simulink model "vrcrane_traj"  (Simulink 6.0)
settings: Solver=ode45  StartTime=0.0  StopTime=60  RelTol=1e-3
PostLoadFcn:
  | Ra=2.6;
  | La=0.012;
  | B=1e-1;
  | Kt=1e2;
  | Kv=3e-2;
  | Kg=1e-3;
  | J=0.1;
  | g=9.80665;
  | m_head=100;
  | Gamma=10;
undefined symbols (not defined in the file or in its folder): sigbuilder_block
libraries: simulink_extras x6, vrlib x6, simulink x1
settings Model: Creator=Danek  LastModifiedBy=Danek
settings DataIOCC: SignalLoggingName=logsOut
settings DebuggingCC: CheckExecutionContextPreStartOutputMsg=on  CheckExecutionContextRuntimeOutputMsg=on
settings ModelReferenceCC: UpdateModelReferenceTargets=IfOutOfDate
settings GRTTargetCC: LifeSpan=inf
settings SFSimCC: SFSimApplyToAllLibs=on  SFSimBuildMode=Incremental

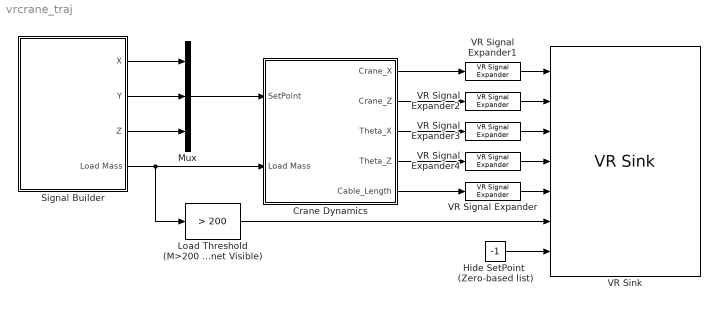
== system vrcrane_traj ==
  Crane Dynamics : Subsystem  EnableExecutionContextPropagation=on
  Hide SetPoint  (Zero-based list) : Constant  Value=-1
  Load Threshold (M>200 = Load on Magnet Visible) : simulink/Logic and Bit Operations/Compare To Constant  relop=>  const=200  LogicOutDataTypeMode=uint8
  Mux : Mux  Inputs=3
  Signal Builder : Subsystem  Tag=STV Subsys  LoadFcn=sigbuilder_block('load');  StartFcn=sigbuilder_block('start');  StopFcn=sigbuilder_block('stop');  ClipboardFcn=sigbuilder_block('clipboard');  EnableExecutionContextPropagation=on  mask(Sigbuilder block){}
      mask help: Sigbuilder GUI
      mask init:
      | if ~strcmp(get_param(bdroot(gcb),'SimulationStatus'),'stopped') tuvar = sigbuilder_block('maskInit'); end
      settings: CopyFcn=sigbuilder_block('copy');  DeleteFcn=sigbuilder_block('delete');  ModelCloseFcn=sigbuilder_block('modelClose');  PreSaveFcn=sigbuilder_block('preSave');  NameChangeFcn=sigbuilder_block('namechange');  OpenFcn=sigbuilder_block('open',[111.75 57.75 534.75 459.75 ]);  CloseFcn=sigbuilder_block('close');
      mask Display: plot(0,0,100,100,[10,10,40,40,10],[80,20,20,80,80],[40,10],[50,50], [40,27,10],[65,72,56],[40,25,25,10],[28,28,43,43]);
  VR Signal Expander : vrlib/VR Signal Expander  outwidth=3  outidx=[2]
  VR Signal Expander1 : vrlib/VR Signal Expander  outwidth=3  outidx=[1]
  VR Signal Expander2 : vrlib/VR Signal Expander  outwidth=3  outidx=[3]
  VR Signal Expander3 : vrlib/VR Signal Expander  outwidth=4  outidx=[4]
  VR Signal Expander4 : vrlib/VR Signal Expander  outwidth=4  outidx=[4]
  VR Sink : vrlib/VR Sink  SampleTime=0.1  ViewEnable=on  RemoteChange=off  RemoteView=off  FieldsWritten=Crane_X.translation.3.1.double#Crane_Z.translation.3.1.double#Parts_Rot_ZAxis.rotation.4.1.double#Parts_Rot_XAxis.rotation.4.1.double#CableUnit.scale.3.1.double#Load_Switch.whichChoice.1.1.double#SP_Highlight.whichChoice.1.1.double  WorldFileName=portal_crane.wrl  WorldDescription=VR Portal Crane  AutoView=on  FigureProperties="{'Position', 'Name', 'Viewpoint', 'CameraBound', 'CameraDirection', 'CameraPosition', 'CameraUpVector', 'ZoomFactor', 'Antialiasing', 'Headlight', 'Lighting', 'NavPanel', 'StatusBar', 'Textures', 'Transparency', 'Wireframe', 'NavZones', 'NavMode', 'NavSpeed', 'Record2DCompressMethod', 'Record2DCompressQuality', 'Record2D', 'Record2DFcn', 'Record2DFileName', 'Record2DStartFcn', 'Record2DStopFcn'; [1.3000000000000000e+001  7.8000000000000000e+001  5.7600000000000000e+002  3.8000000000000000e+002], 'VR Portal Crane', 'Overview', 'on', [-4.7942553860420378e-001  2.7565528915671302e-002 -8.7714952804505797e-001], [8.7686886571229490e+000 -3.9860053732208831e+000 -2.1939948026302826e+001], [3.4694469519536142e-017  9.9950656056293841e-001  3.1410752802896708e-002], [1.0000000000000000e+000], 'off', 'on', 'on', 'halfbar', 'on', 'on', 'on', 'off', 'off', 'examine', 'normal', 'auto', [7.5000000000000000e+001], 'off', 'vrrecordcallback(vrgcbf, ''Frame'');', '%f_anim_%n.avi', 'vrrecordcallback(vrgcbf, ''Start'');', 'vrrecordcallback(vrgcbf, ''Stop'');'}"
  wires:
  Crane Dynamics/5(Cable_Length) -> VR Signal Expander/1
  Crane Dynamics/1(Crane_X) -> VR Signal Expander1/1
  Crane Dynamics/3(Theta_X) -> VR Signal Expander3/1
  Crane Dynamics/2(Crane_Z) -> VR Signal Expander2/1
  Crane Dynamics/4(Theta_Z) -> VR Signal Expander4/1
  Mux/1 -> Crane Dynamics/1(SetPoint)
  Signal Builder/1(X) -> Mux/1
  Signal Builder/2(Y) -> Mux/2
  Signal Builder/3(Z) -> Mux/3
  Signal Builder/4(Load Mass) -> Crane Dynamics/2(Load Mass), Load Threshold (M>200 = Load on Magnet Visible)/1
  VR Signal Expander1/1 -> VR Sink/1
  VR Signal Expander2/1 -> VR Sink/2
  VR Signal Expander3/1 -> VR Sink/3
  VR Signal Expander4/1 -> VR Sink/4
  VR Signal Expander/1 -> VR Sink/5
  Load Threshold (M>200 = Load on Magnet Visible)/1 -> VR Sink/6
  Hide SetPoint  (Zero-based list)/1 -> VR Sink/7

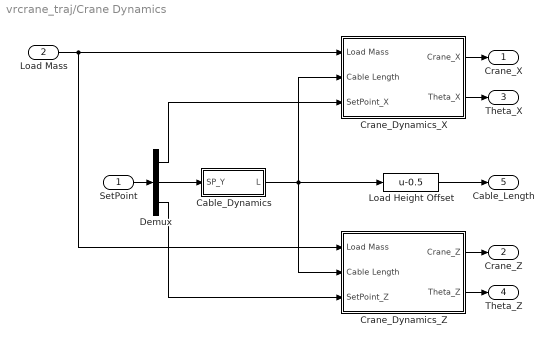
== system vrcrane_traj/Crane Dynamics ==
  SetPoint : Inport  LatchInput=off
  Load Mass : Inport  Port=2  LatchInput=off
  Cable_Dynamics : Subsystem  EnableExecutionContextPropagation=on
  Crane_Dynamics_X : Subsystem  EnableExecutionContextPropagation=on
  Crane_Dynamics_Z : Subsystem  EnableExecutionContextPropagation=on
  Demux : Demux  Outputs=3
  "Load Height Offset " : Fcn  Expr=u-0.5
  Crane_X : Outport
  Crane_Z : Outport  Port=2
  Theta_X : Outport  Port=3
  Theta_Z : Outport  Port=4
  Cable_Length : Outport  Port=5
  wires:
  Cable_Dynamics/1(L) -> Crane_Dynamics_X/2(Cable Length), Crane_Dynamics_Z/2(Cable Length), "Load Height Offset "/1
  Demux/2 -> Cable_Dynamics/1(SP_Y)
  Demux/1 -> Crane_Dynamics_X/3(SetPoint_X)
  Load Mass/1 -> Crane_Dynamics_Z/1(Load Mass), Crane_Dynamics_X/1(Load Mass)
  SetPoint/1 -> Demux/1
  Crane_Dynamics_X/1(Crane_X) -> Crane_X/1
  Crane_Dynamics_X/2(Theta_X) -> Theta_X/1
  "Load Height Offset "/1 -> Cable_Length/1
  Crane_Dynamics_Z/1(Crane_Z) -> Crane_Z/1
  Crane_Dynamics_Z/2(Theta_Z) -> Theta_Z/1
  Demux/3 -> Crane_Dynamics_Z/3(SetPoint_Z)

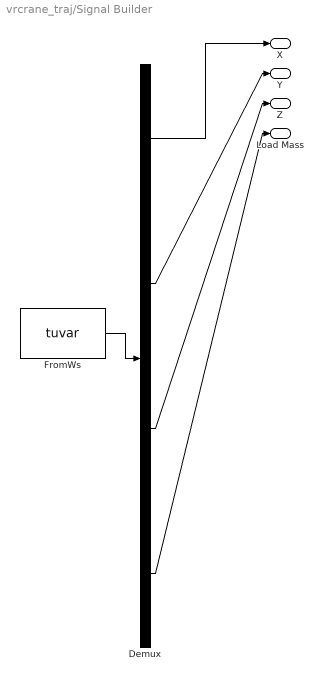
== system vrcrane_traj/Signal Builder ==
  Demux : Demux  Tag=STV Demux
  FromWs : FromWorkspace  Tag=STV FromWs  VariableName=tuvar  SampleTime=0  OutputAfterFinalValue=Holding final value  SigBuilderData=DataTag0  VnvData=DataTag1
      SigBuilderData=|
      | channels(1).label = 'X'
      | channels(1).allXData = {[0 17.9 17.9 34.9 34.9 35 36.8 36.8 60]}
      | channels(1).allYData = {[0 0 15 15 15.5 15 15 0 0]}
      | channels(2).label = 'Y'
      | channels(2).allXData = {[0 14 14 18 18 32 32 35 36.8 36.8 50 50 60]}
      | channels(2).allYData = {[4 4 0 0 4 4 0 0 0 4 4 0 0]}
      | channels(3).label = 'Z'
      | channels(3).allXData = {[0 3 3 18 18 34.9 35 37 37 60]}
      | channels(3).allYData = {[0 0 15 15 5 5 5 5 0 0]}
      | channels(4).label = 'Load Mass'
      | channels(4).allXData = {[0 17 17 36.2 36.2 60]}
      | channels(4).allYData = {[100 100 1000 1000 100 100]}
      | common.afterFinalStr = 'Hold final value'
      | common.sampleTime = 0
      | dataSet.timeRange = [0 60]
      | dataSet.name = 'Setpoint'
  X : Outport  Tag=STV Outport
  Y : Outport  Tag=STV Outport  Port=2
  Z : Outport  Tag=STV Outport  Port=3
  Load Mass : Outport  Tag=STV Outport  Port=4
  wires:
  Demux/1 -> X/1
  FromWs/1 -> Demux/1
  Demux/2 -> Y/1
  Demux/3 -> Z/1
  Demux/4 -> Load Mass/1

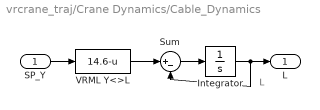
== system vrcrane_traj/Crane Dynamics/Cable_Dynamics ==
  note: L
  SP_Y : Inport  LatchInput=off
  Integrator : Integrator  InitialCondition=14.6  LimitOutput=on  UpperSaturationLimit=14.6  LowerSaturationLimit=4.6
  Sum : Sum  Inputs=|+-
  VRML Y<>L : Fcn  Expr=14.6-u
  L : Outport
  wires:
  Sum/1 -> Integrator/1
  VRML Y<>L/1 -> Sum/1
  Integrator/1 -> Sum/2, L/1
  SP_Y/1 -> VRML Y<>L/1

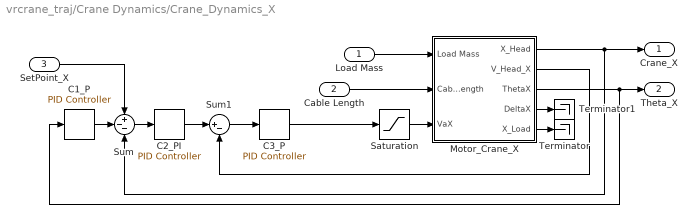
== system vrcrane_traj/Crane Dynamics/Crane_Dynamics_X ==
  Load Mass : Inport  LatchInput=off
  Cable Length : Inport  Port=2  LatchInput=off
  SetPoint_X : Inport  Port=3  LatchInput=off
  C1_P : simulink_extras/Additional Linear/PID Controller  P=-20  I=0  D=0
  C2_PI : simulink_extras/Additional Linear/PID Controller  P=2.5  I=0  D=0
  C3_P : simulink_extras/Additional Linear/PID Controller  P=5  I=0  D=0
  Motor_Crane_X : Subsystem  EnableExecutionContextPropagation=on
  Saturation : Saturate  UpperLimit=50  LowerLimit=-50
  Sum : Sum  Inputs=+--  SaturateOnIntegerOverflow=on  InputSameDT=on
  Sum1 : Sum  Inputs=|+-  SaturateOnIntegerOverflow=on  InputSameDT=on
  Terminator : Terminator
  Terminator1 : Terminator
  Crane_X : Outport
  Theta_X : Outport  Port=2
  wires:
  Motor_Crane_X/1(X_Head) -> Crane_X/1, Sum/3
  Load Mass/1 -> Motor_Crane_X/1(Load Mass)
  Motor_Crane_X/2(V_Head_X) -> Sum1/2
  Cable Length/1 -> Motor_Crane_X/2(Cable Length)
  Motor_Crane_X/3(ThetaX) -> Theta_X/1, C1_P/1
  Motor_Crane_X/4(DeltaX) -> Terminator1/1
  Motor_Crane_X/5(X_Load) -> Terminator/1
  SetPoint_X/1 -> Sum/1
  Sum/1 -> C2_PI/1
  C2_PI/1 -> Sum1/1
  Sum1/1 -> C3_P/1
  Saturation/1 -> Motor_Crane_X/3(VaX)
  C3_P/1 -> Saturation/1
  C1_P/1 -> Sum/2

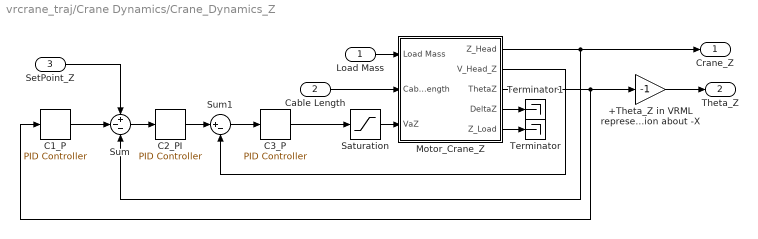
== system vrcrane_traj/Crane Dynamics/Crane_Dynamics_Z ==
  Load Mass : Inport  LatchInput=off
  Cable Length : Inport  Port=2  LatchInput=off
  SetPoint_Z : Inport  Port=3  LatchInput=off
  +Theta_Z in VRML represented by rotation about -X : Gain  Gain=-1
  C1_P : simulink_extras/Additional Linear/PID Controller  P=-20  I=0  D=0
  C2_PI : simulink_extras/Additional Linear/PID Controller  P=2.5  I=0  D=0
  C3_P : simulink_extras/Additional Linear/PID Controller  P=5  I=0  D=0
  Motor_Crane_Z : Subsystem  EnableExecutionContextPropagation=on
  Saturation : Saturate  UpperLimit=50  LowerLimit=-50
  Sum : Sum  Inputs=+--  SaturateOnIntegerOverflow=on  InputSameDT=on
  Sum1 : Sum  Inputs=|+-  SaturateOnIntegerOverflow=on  InputSameDT=on
  Terminator : Terminator
  Terminator1 : Terminator
  Crane_Z : Outport
  Theta_Z : Outport  Port=2
  wires:
  Motor_Crane_Z/1(Z_Head) -> Crane_Z/1, Sum/3
  Load Mass/1 -> Motor_Crane_Z/1(Load Mass)
  Cable Length/1 -> Motor_Crane_Z/2(Cable Length)
  Motor_Crane_Z/3(ThetaZ) -> +Theta_Z in VRML represented by rotation about -X/1, C1_P/1
  Motor_Crane_Z/4(DeltaZ) -> Terminator1/1
  Motor_Crane_Z/5(Z_Load) -> Terminator/1
  Saturation/1 -> Motor_Crane_Z/3(VaZ)
  C3_P/1 -> Saturation/1
  +Theta_Z in VRML represented by rotation about -X/1 -> Theta_Z/1
  Motor_Crane_Z/2(V_Head_Z) -> Sum1/2
  Sum/1 -> C2_PI/1
  C2_PI/1 -> Sum1/1
  Sum1/1 -> C3_P/1
  C1_P/1 -> Sum/2
  SetPoint_Z/1 -> Sum/1

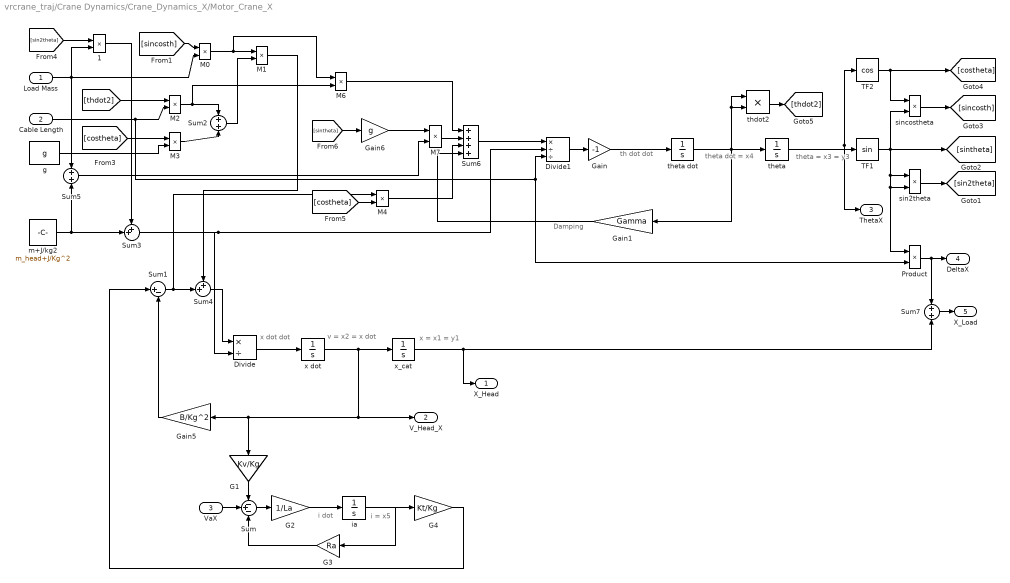
== system vrcrane_traj/Crane Dynamics/Crane_Dynamics_X/Motor_Crane_X ==
  note: i dot
  note: i = x5
  note: x = x1 = y1
  note: v = x2 = x dot
  note: theta = x3 = y3
  note: theta dot = x4
  note: x dot dot
  note: th dot dot
  note: Damping
  Load Mass : Inport  LatchInput=off
  Cable Length : Inport  Port=2  LatchInput=off
  VaX : Inport  Port=3  LatchInput=off
  " 1" : Product  Inputs=**  OutScaling=2^-10
  Divide : Product  Inputs=*/  OutScaling=2^-10
  Divide1 : Product  Inputs=*//  OutScaling=2^-10
  G1 : Gain  Orientation=down  Gain=Kv/Kg
  G2 : Gain  Gain=1/La
  G3 : Gain  Orientation=left  Gain=Ra
  G4 : Gain  Gain=Kt/Kg
  Gain : Gain  Gain=-1
  Gain1 : Gain  Orientation=left  Gain=Gamma
  Gain5 : Gain  Orientation=left  Gain=B/Kg^2
  Gain6 : Gain  Gain=g
  M{0..4,6..7} (7 alike) : Product  Inputs=**  OutScaling=2^-10
  Product : Product  SaturateOnIntegerOverflow=on
  Sum : Sum  Inputs=-+-
  Sum1 : Sum  Inputs=|+-
  Sum2 : Sum
  Sum3 : Sum  Inputs=++|
  Sum4 : Sum  Inputs=++|
  Sum5 : Sum
  Sum6 : Sum  Inputs=++++
  Sum7 : Sum
  TF1 : Trigonometry
  TF2 : Trigonometry  Operator=cos
  g : Constant  Value=g
  ia : Integrator
  m+J/kg2 : Constant  Value=m_head+J/Kg^2
  sin2theta : Product  Inputs=**  OutScaling=2^-10
  sincostheta : Product  Inputs=**  OutScaling=2^-10
  thdot2 : Product  Inputs=**  OutScaling=2^-10
  theta : Integrator
  theta dot : Integrator
  x dot : Integrator
  x_cat : Integrator
  X_Head : Outport
  V_Head_X : Outport  Port=2
  ThetaX : Outport  Port=3
  DeltaX : Outport  Port=4
  X_Load : Outport  Port=5
  wires:
  G1/1 -> Sum/1
  Sum/1 -> G2/1
  G2/1 -> ia/1
  ia/1 -> G3/1, G4/1
  G3/1 -> Sum/3
  x dot/1 -> x_cat/1, G1/1, Gain5/1, V_Head_X/1
  theta/1 -> ThetaX/1, TF1/1, TF2/1
  theta dot/1 -> theta/1, thdot2/2, thdot2/1, Gain1/1
  G4/1 -> Sum1/1
  Divide/1 -> x dot/1
  Gain5/1 -> Sum1/2
  sin2theta/1 -> [sin2theta]
  sincostheta/1 -> [sincosth]
  [sincosth] -> M0/1
  Load Mass/1 -> Sum5/1, M0/2, " 1"/2
  thdot2/1 -> [thdot2]
  M0/1 -> M1/1, M6/1
  [thdot2] -> M2/1
  [costheta] -> M3/1
  g/1 -> M3/2
  M3/1 -> Sum2/2
  Sum2/1 -> M1/2
  [sin2theta] -> " 1"/1
  " 1"/1 -> Sum3/1
  Sum3/1 -> Divide1/2, Divide/2
  Sum4/1 -> Divide/1
  M1/1 -> Sum4/1
  Sum1/1 -> Sum4/2, M4/1
  M2/1 -> Sum2/1, M6/2
  M6/1 -> Sum6/1
  [costheta] -> M4/2
  Sum5/1 -> M7/2
  [sintheta] -> Gain6/1
  Gain6/1 -> M7/1
  M7/1 -> Sum6/2
  M4/1 -> Sum6/3
  Sum6/1 -> Divide1/1
  Cable Length/1 -> M2/2, Divide1/3, Product/2
  Divide1/1 -> Gain/1
  Gain/1 -> theta dot/1
  x_cat/1 -> X_Head/1, Sum7/2
  VaX/1 -> Sum/2
  m+J/kg2/1 -> Sum3/2, Sum5/2
  Product/1 -> DeltaX/1, Sum7/1
  TF2/1 -> [costheta], sincostheta/1
  TF1/1 -> [sintheta], sincostheta/2, sin2theta/2, Product/1, sin2theta/1
  Sum7/1 -> X_Load/1
  Gain1/1 -> Sum6/4

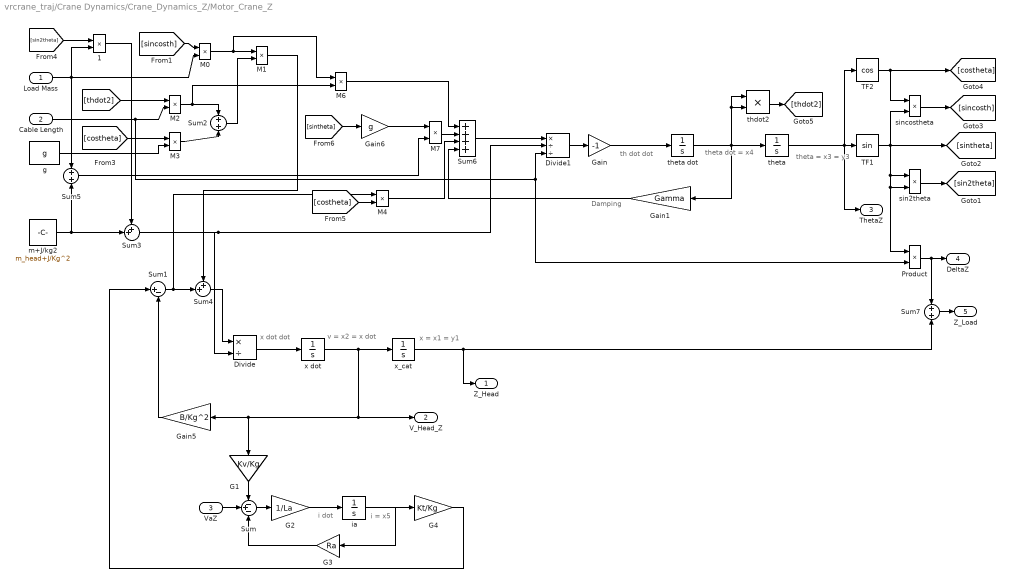
== system vrcrane_traj/Crane Dynamics/Crane_Dynamics_Z/Motor_Crane_Z ==
  note: i dot
  note: i = x5
  note: x = x1 = y1
  note: v = x2 = x dot
  note: theta = x3 = y3
  note: theta dot = x4
  note: x dot dot
  note: th dot dot
  note: Damping
  Load Mass : Inport  LatchInput=off
  Cable Length : Inport  Port=2  LatchInput=off
  VaZ : Inport  Port=3  LatchInput=off
  " 1" : Product  Inputs=**  OutScaling=2^-10
  Divide : Product  Inputs=*/  OutScaling=2^-10
  Divide1 : Product  Inputs=*//  OutScaling=2^-10
  G1 : Gain  Orientation=down  Gain=Kv/Kg
  G2 : Gain  Gain=1/La
  G3 : Gain  Orientation=left  Gain=Ra
  G4 : Gain  Gain=Kt/Kg
  Gain : Gain  Gain=-1
  Gain1 : Gain  Orientation=left  Gain=Gamma
  Gain5 : Gain  Orientation=left  Gain=B/Kg^2
  Gain6 : Gain  Gain=g
  M{0..4,6..7} (7 alike) : Product  Inputs=**  OutScaling=2^-10
  Product : Product  SaturateOnIntegerOverflow=on
  Sum : Sum  Inputs=-+-
  Sum1 : Sum  Inputs=|+-
  Sum2 : Sum
  Sum3 : Sum  Inputs=++|
  Sum4 : Sum  Inputs=++|
  Sum5 : Sum
  Sum6 : Sum  Inputs=++++
  Sum7 : Sum
  TF1 : Trigonometry
  TF2 : Trigonometry  Operator=cos
  g : Constant  Value=g
  ia : Integrator
  m+J/kg2 : Constant  Value=m_head+J/Kg^2
  sin2theta : Product  Inputs=**  OutScaling=2^-10
  sincostheta : Product  Inputs=**  OutScaling=2^-10
  thdot2 : Product  Inputs=**  OutScaling=2^-10
  theta : Integrator
  theta dot : Integrator
  x dot : Integrator
  x_cat : Integrator
  Z_Head : Outport
  V_Head_Z : Outport  Port=2
  ThetaZ : Outport  Port=3
  DeltaZ : Outport  Port=4
  Z_Load : Outport  Port=5
  wires:
  G1/1 -> Sum/1
  Sum/1 -> G2/1
  G2/1 -> ia/1
  ia/1 -> G3/1, G4/1
  G3/1 -> Sum/3
  x dot/1 -> x_cat/1, G1/1, Gain5/1, V_Head_Z/1
  theta/1 -> ThetaZ/1, TF1/1, TF2/1
  theta dot/1 -> theta/1, thdot2/2, thdot2/1, Gain1/1
  G4/1 -> Sum1/1
  Divide/1 -> x dot/1
  Gain5/1 -> Sum1/2
  sin2theta/1 -> [sin2theta]
  sincostheta/1 -> [sincosth]
  [sincosth] -> M0/1
  Load Mass/1 -> Sum5/1, M0/2, " 1"/2
  thdot2/1 -> [thdot2]
  M0/1 -> M1/1, M6/1
  [thdot2] -> M2/1
  [costheta] -> M3/1
  g/1 -> M3/2
  M3/1 -> Sum2/2
  Sum2/1 -> M1/2
  [sin2theta] -> " 1"/1
  " 1"/1 -> Sum3/1
  Sum3/1 -> Divide1/2, Divide/2
  Sum4/1 -> Divide/1
  M1/1 -> Sum4/1
  Sum1/1 -> Sum4/2, M4/1
  M2/1 -> Sum2/1, M6/2
  M6/1 -> Sum6/1
  [costheta] -> M4/2
  Sum5/1 -> M7/2
  [sintheta] -> Gain6/1
  Gain6/1 -> M7/1
  M7/1 -> Sum6/2
  M4/1 -> Sum6/3
  Sum6/1 -> Divide1/1
  Cable Length/1 -> M2/2, Divide1/3, Product/2
  Divide1/1 -> Gain/1
  Gain/1 -> theta dot/1
  x_cat/1 -> Z_Head/1, Sum7/2
  VaZ/1 -> Sum/2
  m+J/kg2/1 -> Sum3/2, Sum5/2
  Product/1 -> DeltaZ/1, Sum7/1
  TF2/1 -> [costheta], sincostheta/1
  TF1/1 -> [sintheta], sincostheta/2, sin2theta/2, Product/1, sin2theta/1
  Sum7/1 -> Z_Load/1
  Gain1/1 -> Sum6/4
